simulink model "sdruFMStereoMidi"  (R2014a)
settings: Solver=FixedStepDiscrete  SolverMode=SingleTasking  StartTime=0.0  StopTime=inf  RelTol=1e-3
PreLoadFcn:
  | stereoFM = getParamsSdruFMStereoDemo;
InitFcn:
  | stereoFM = getParamsSdruFMStereoDemo;
undefined symbols (not defined in the file or in its folder): mfilt, Normalized
libraries: dspmlti4 x2, dsparch4 x2, dspsnks4 x1, dspsigops x1, simulink x1, sdrublksprivate x1, dspsrcs4 x1, commsdrhw_v2 x1
CloseFcn:
  | clear stereoFM
Description:
  | This model uses Universal Software Radio Peripheral (USRP) hardware with Simulink(R) to perform FM demodulation and stereo decoding.
settings Model: Creator=The MathWorks Inc.
settings DataIOCC: LimitDataPoints=off  SaveFormat=Structure  SignalLoggingSaveFormat=ModelDataLogs  SaveOutput=off  SignalLogging=off  DSMLogging=off  SaveTime=off
settings OptimizationCC: ExpressionDepthLimit=2147483647  EfficientMapNaN2IntZero=off  SimCompilerOptimization=On
settings DebuggingCC: UnderspecifiedInitializationDetection=Classic  InheritedTsInSrcMsg=none  MultiTaskCondExecSysMsg=none  ParameterPrecisionLossMsg=none  FcnCallInpInsideContextMsg=UseLocalSettings  StateNameClashWarn=warning
settings HardwareCC: TargetBitPerLong=64  TargetBitPerPointer=64  TargetLongLongMode=on  TargetIntDivRoundTo=Zero  TargetEndianess=LittleEndian  TargetWordSize=64  TargetHWDeviceType=Generic->MATLAB Host Computer  ProdEqTarget=off
settings SFSimCC: SFSimEnableDebug=off  SFSimOverflowDetection=off  SimIntegrity=off
settings RTWCC: CustomSourceCode=|
  | #include <stdio.h>
  | #include <stdlib.h>
settings CodeAppCC: MaxIdLength=128
settings GRTTargetCC: CombineOutputUpdateFcns=off  GRTInterface=on

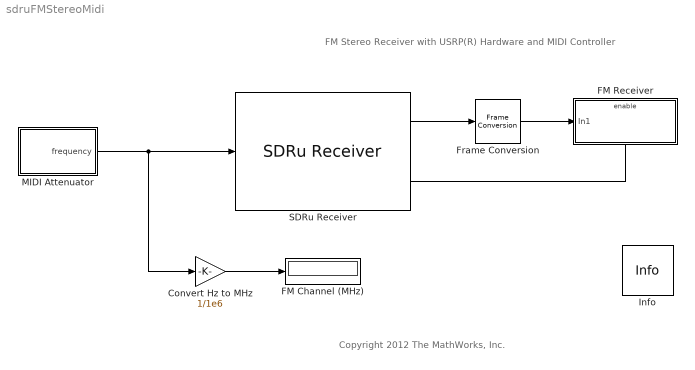
== system sdruFMStereoMidi ==
  note: Copyright 2012 The MathWorks, Inc.
  note: FM Stereo Receiver with USRP(R) Hardware and MIDI Controller
  "Convert Hz to MHz " : Gain  Gain=1/1e6
  FM Channel (MHz) : Display
  FM Receiver : Subsystem  TreatAsAtomicUnit=on
  Frame Conversion : FrameConversion
  Info : sdrublksprivate/Info  SystemSampleTime=-1
  MIDI Attenuator : Subsystem  mask{UseSpecifiedDevice=Default, DeviceName='', UseSpecifiedControls=Respond to any control, ControlNumbers=0}
      mask prompts: UseSpecifiedDevice "MIDI Device:"; DeviceName "MIDI device name:"; UseSpecifiedControls "MIDI controls:"; ControlNumbers "MIDI control numbers:"
      mask init:
      | set_param([gcb '/MIDI Controls'], 'UseSpecifiedDevice', get_param(gcb,'UseSpecifiedDevice'));
      | set_param([gcb '/MIDI Controls'], 'UseSpecifiedControls', get_param(gcb,'UseSpecifiedControls'));
      mask TypeOptions UseSpecifiedDevice: Default | Specify other
      mask Callback UseSpecifiedDevice:
      | switch 2*~isempty(strfind(get_param(gcbh,'UseSpecifiedDevice'),'pecif')) ...
      |         + ~isempty(strfind(get_param(gcbh,'UseSpecifiedControls'),'pecif'))
      |     case 0
      |         set_param(gcbh,'MaskVisibilities',{'on','off','on','off'});
      |     case 1
      |         set_param(gcbh,'MaskVisibilities',{'on','off','on','on'});
      |     case 2
      |         set_param(gcbh,'MaskVisibilities',{'on','on','on','off'});
      |     case 3
      |         set_param(gcbh,'MaskVisibilities',{'on','on','on','on'});
      | end
      mask TypeOptions DeviceName: MIDI Controls/DeviceName
      mask TypeOptions UseSpecifiedControls: Respond to any control | Respond to specified controls
      mask Callback UseSpecifiedControls:
      | switch 2*~isempty(strfind(get_param(gcbh,'UseSpecifiedDevice'),'pecif')) ...
      |         + ~isempty(strfind(get_param(gcbh,'UseSpecifiedControls'),'pecif'))
      |     case 0
      |         set_param(gcbh,'MaskVisibilities',{'on','off','on','off'});
      |     case 1
      |         set_param(gcbh,'MaskVisibilities',{'on','off','on','on'});
      |     case 2
      |         set_param(gcbh,'MaskVisibilities',{'on','on','on','off'});
      |     case 3
      |         set_param(gcbh,'MaskVisibilities',{'on','on','on','on'});
      | end
      mask TypeOptions ControlNumbers: MIDI Controls/ControlNumbers
      mask Display: disp('MIDI Station\nSelector')
  SDRu Receiver : commsdrhw_v2/SDRu Receiver  rxtx=rx  USRP2_IP='192.168.10.2'  centerFrequency=2.45e9  centerFrequencySrc=Input port  loOffset=0  loOffsetSrc=Dialog  gain=stereoFM.USRPGain  gainSrc=Dialog  decimInterp=stereoFM.USRPDecimationFactor  decimInterpSrc=Dialog  USRP2_IP_NUM=[49 57 50 46 49 54 56 46 49 48 46 50]  frameLength=stereoFM.FrameLength  outputDatatype=single  overrunUnderrunPort=off  sampleTime=1/(100e6/stereoFM.USRPDecimationFactor)  HOST_DATA_PORT=30000  HOST_CONTROL_PORT=30002  USRP2_DATA_PORT=32769  USRP2_CONTROL_PORT=32768  bufferMode=Continuous streaming  EnableBurstMode=off  NumFramesInBurst=100
  wires:
  SDRu Receiver/1 -> Frame Conversion/1
  SDRu Receiver/2 -> FM Receiver/Enable
  Frame Conversion/1 -> FM Receiver/1(In1)
  MIDI Attenuator/1(frequency) -> SDRu Receiver/1, "Convert Hz to MHz "/1
  "Convert Hz to MHz "/1 -> FM Channel (MHz)/1

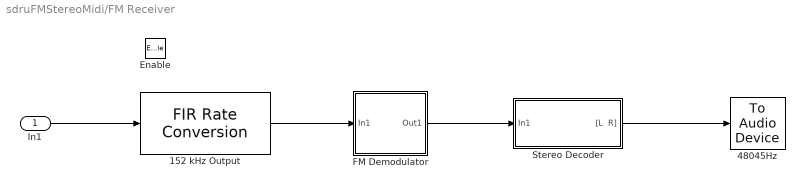
== system sdruFMStereoMidi/FM Receiver ==
  In1 : Inport
  Enable : EnablePort
  152 kHz Output : dspmlti4/FIR Rate Conversion  L=136  h=[9]  M=179  firstCoeffDataTypeStr=Inherit: Same word length as input  firstCoeffLastDataTypeStr=Inherit: Same word length as input  firstCoeffMin=[]  firstCoeffMax=[]  outputDataTypeStr=Inherit: Same as accumulator  outputLastDataTypeStr=Inherit: Same as accumulator  outputMin=[]  outputMax=[]  roundingMode=Floor  overflowMode=off  FilterSource=Filter object  FilterObject=mfilt.firsrc(stereoFM.RCDemodInterpFactor,stereoFM.RCDemodDecimFactor)
  48045Hz : dspsnks4/To Audio Device  deviceName=Default  inheritSampleRate=on  sampleRate=48045  deviceDatatype=Determine from input data type  autoBufferSize=on  bufferSize=4096  queueDuration=1.0  defaultOutputChannelMapping=on  outputChannelMapping=1
  "FM Demodulator " : Subsystem
      mask Display: disp('FM\nDemodulator')
  Stereo Decoder : Subsystem
  wires:
  Stereo Decoder/1("[L  R]") -> 48045Hz/1
  152 kHz Output/1 -> "FM Demodulator "/1(In1)
  "FM Demodulator "/1(Out1) -> Stereo Decoder/1(In1)
  In1/1 -> 152 kHz Output/1

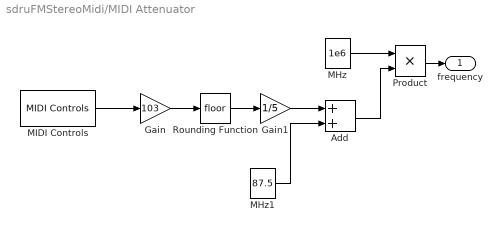
== system sdruFMStereoMidi/MIDI Attenuator ==
  Add : Sum
  Gain : Gain  Gain=103
  Gain1 : Gain  Gain=1/5
  MHz : Constant  Value=1e6  VectorParams1D=off  SampleTime=-1  FramePeriod=-1
  MHz1 : Constant  Value=87.5  VectorParams1D=off  SampleTime=-1  FramePeriod=-1
  MIDI Controls : dspsrcs4/MIDI Controls  UseSpecifiedDevice=Default  DeviceName=DeviceName  UseSpecifiedControls=Respond to any control  ControlNumbers=ControlNumbers  InitialValues=0.735  SyncAtStart=off  RawUint8=Normalized (0 - 1)
  Product : Product  RndMeth=Zero
  Rounding Function : Rounding
  frequency : Outport
  wires:
  MHz/1 -> Product/1
  MHz1/1 -> Add/2
  Product/1 -> frequency/1
  Add/1 -> Product/2
  Gain/1 -> Rounding Function/1
  Rounding Function/1 -> Gain1/1
  Gain1/1 -> Add/1
  MIDI Controls/1 -> Gain/1

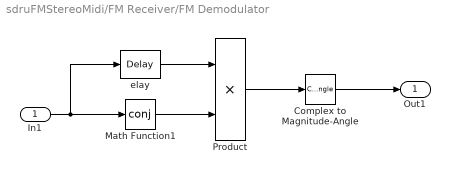
== system sdruFMStereoMidi/FM Receiver/FM Demodulator  ==
  In1 : Inport
  Complex to Magnitude-Angle : ComplexToMagnitudeAngle  Output=Angle
  Math Function1 : Math  Operator=conj  SaturateOnIntegerOverflow=on
  Product : Product  RndMeth=Zero
  elay : dspsigops/Delay  InputProcessing=Columns as channels (frame based)  dly_unit=Samples  delay=1  ic_detail=off  dif_ic_for_ch=off  dif_ic_for_dly=off  ic=0  reset_popup=None
  Out1 : Outport
  wires:
  Math Function1/1 -> Product/2
  Product/1 -> Complex to Magnitude-Angle/1
  elay/1 -> Product/1
  Complex to Magnitude-Angle/1 -> Out1/1
  In1/1 -> Math Function1/1, elay/1

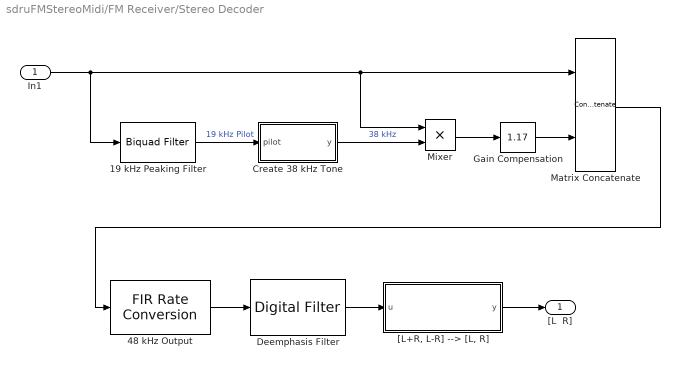
== system sdruFMStereoMidi/FM Receiver/Stereo Decoder ==
  In1 : Inport
  19 kHz Peaking Filter : dsparch4/Biquad Filter  IIRFiltStruct=Direct form II  CoeffSource=Specify via dialog  BiQuadCoeffs=[1 1 1 1 1 1]  a0Flag=Warning  IC=0  ICnum=0  ICden=0  InputProcessing=Columns as channels (frame based)  denAccumFracLength=30  denProdOutputFracLength=30  secondMemoryFracLength=15  roundingMode=Floor  overflowMode=off  ScaleValues=1  optimizeScaleValues=on  ScaleValueMode=Specify via input port (g)  scaleValueFracLength=14  FilterSource=dfilt object  dfiltObjectName=stereoFM.peak19fil
  48 kHz Output : dspmlti4/FIR Rate Conversion  L=stereoFM.RCAudioInterpFactor  h=stereoFM.LP15k  M=stereoFM.RCAudioDecimFactor  firstCoeffDataTypeStr=Inherit: Same word length as input  firstCoeffLastDataTypeStr=Inherit: Same word length as input  firstCoeffMin=[]  firstCoeffMax=[]  outputDataTypeStr=Inherit: Same as accumulator  outputLastDataTypeStr=Inherit: Same as accumulator  outputMin=[]  outputMax=[]  roundingMode=Floor  overflowMode=off  FilterSource=Specify via dialog  FilterObject=MFobj4n
  Create 38 kHz Tone : MATLAB Function  TreatAsAtomicUnit=on
  Deemphasis Filter : dsparch4/Digital Filter  TypePopup=IIR (poles & zeros)  IIRFiltStruct=Biquad direct form I (SOS)  AllPoleFiltStruct=Direct form  FIRFiltStruct=Direct form  CoeffSource=Specify via dialog  NumCoeffs=[1 2]  DenCoeffs=[1 0.1]  BiQuadCoeffs=[1 1 1 1 1 1]  LatticeCoeffs=[0.2 0.4]  denIgnore=on  FiltPerSampPopup=One filter per frame  IC=0  ICnum=0  ICden=0  roundingMode=Floor  overflowMode=off  ScaleValues=1  scaleValueFracLength=14  stageInFracLength=15  stageOutFracLength=15  FilterSource=dfilt object  dfiltObjectName=stereoFM.Deemp  InputProcessing=Columns as channels (frame based)
  Gain Compensation : simulink/Math Operations/Slider Gain  low=0  gain=1.17  high=10
  Matrix Concatenate : Concatenate  Mode=Multidimensional array  ConcatenateDimension=2
  Mixer : Product  RndMeth=Zero
  "[L+R, L-R] --> [L, R]" : MATLAB Function  TreatAsAtomicUnit=on
  "[L  R]" : Outport
  wires:
  In1/1 -> 19 kHz Peaking Filter/1, Mixer/1, Matrix Concatenate/1
  19 kHz Peaking Filter/1 -> Create 38 kHz Tone/1(pilot)  "19 kHz Pilot"
  Create 38 kHz Tone/1(y) -> Mixer/2  "38 kHz"
  48 kHz Output/1 -> Deemphasis Filter/1
  Mixer/1 -> Gain Compensation/1
  Matrix Concatenate/1 -> 48 kHz Output/1
  Deemphasis Filter/1 -> "[L+R, L-R] --> [L, R]"/1(u)
  "[L+R, L-R] --> [L, R]"/1(y) -> "[L  R]"/1
  Gain Compensation/1 -> Matrix Concatenate/2

== matlab function sdruFMStereoMidi/FM Receiver/Stereo Decoder/[L+R, L-R] --> [L, R] ==
  data: u input; y output
function y = StereoSeparation(u)
%#codegen
y = [u(:, 1)+u(:, 2), u(:, 1)-u(:, 2)];

== matlab function sdruFMStereoMidi/FM Receiver/Stereo Decoder/Create 38 kHz Tone ==
  data: pilot input; y output
function y = trig38(pilot)
% Calculate AGC from 19 kHz estimated tone, and apply.
%
% Track max absolute value of latest 8 samples, assuming 152 kHz rate.
% This is our AGC estimate.  Input must be a frame size that is
% a multiple of 8.  Guarantees normalized input never exceeds 1.
%
% Create a phase-locked 38 kHz reference tone for FM demodulation
% based on 19 kHz pilot tone.
%
% To do this, we double the input frequency by use of trigonometric identity
%    sin(2w) = -2 * (-cos(w)) * sin(w)
%


persistent pilot_delay
if isempty(pilot_delay)
    pilot_delay = single(zeros(2,1));
end

%#codegen
y = coder.nullcopy(pilot);  % output frame

N8 = numel(pilot)/8;      % # of 8-sample subframes in input signal
if N8 ~= fix(N8)
    error('Frame size must be a multiple of 8')
end

for idx = 0:N8-1
    % Get next 8 samples from frame
    sidx = idx*8 + 1;
    
    % AGC update
    currMax = max(abs(pilot(sidx:sidx+7)));
    % set minimum currMax to be ~10*eps('single')
    if currMax < eps('single')
        currMax = eps('single');
    end
    
    % Apply AGC
    agc_scale = 1./currMax * sqrt(2);
    
    for j = 0:7
        % AGC is constant over subframe
        % Apply AGC to each subframe samples
        pilot_q = pilot(sidx+j) .* agc_scale; % quadrature term
        
        % Synthesize in-phase from quadrature signal
        % This creates symmetric output (+/- peaks are about equal)
        % For a 19kHz sinusoid at 152kHz sample rate,
        % Delay the sin(w) by two samples, i.e., pi/2 phase shift
        % Obtain -cos(w)
        pilot_i = pilot_delay(2);  % in-phase term
        pilot_delay(2) = pilot_delay(1);
        pilot_delay(1) = pilot_q;
        
        % Create double-freq output from trig identity
        y(sidx+j) = - 2*pilot_q*pilot_i;
    end
end
